simulink model "EMB_Lost_full"  (R2022a)
settings: Solver=VariableStepAuto  StartTime=0.0  StopTime=2  RelTol=1e-3
libraries: slpidlib x24, spsDCVoltageSourceLib x4, spsPermanentMagnetSynchronousMachineLib x4, spsSVPWMGenerator2LevelLib x4, spsUniversalBridgeLib x4, spsdq0toAlphaBetaZeroLib x4, spspowerguiLib x4
(part 1 of 3)
settings Model: SimulationMode=accelerator  Creator=pc  LastModifiedBy=pc

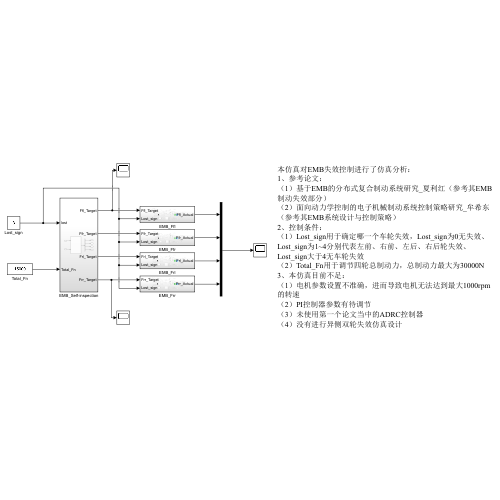
[thumbnail: Simulink's stored preview of the top-level diagram]
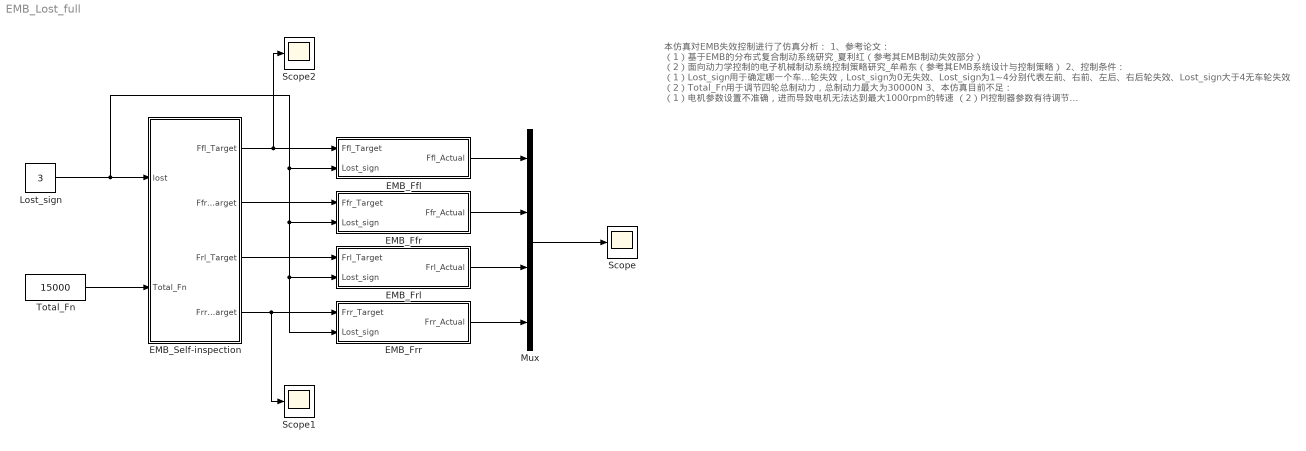
== system EMB_Lost_full ==
  note: 本仿真对EMB失效控制进行了仿真分析：
      | 1、参考论文：
      | （1）基于EMB的分布式复合制动系统研究_夏利红（参考其EMB制动失效部分）
      | （2）面向动力学控制的电子机械制动系统控制策略研究_牟希东（参考其EMB系统设计与控制策略）
      | 2、控制条件：
      | （1）Lost_sign用于确定哪一个车轮失效，Lost_sign为0无失效、Lost_sign为1~4分别代表左前、右前、左后、右后轮失效、Lost_sign大于4无车轮失效
      | （2）Total_Fn用于调节四轮总制动力，总制动力最大为30000N
      | 3、本仿真目前不足：
      | （1）电机参数设置不准确，进而导致电机无法达到最大1000rpm的转速
      | （2）PI控制器参数有待调节
      | （3）未使用第一个论文当中的ADRC控制器
      | （4）没有进行异侧双轮失效仿真设计
  EMB_Ffl : Subsystem
  EMB_Ffr : Subsystem
  EMB_Frl : Subsystem
  EMB_Frr : Subsystem
  EMB_Self-inspection : Subsystem
  Lost_sign : Constant  Value=3
  Mux : Mux
  Scope : Scope
  Scope1 : Scope
  Scope2 : Scope
  Total_Fn : Constant  Value=15000
  wires:
  Total_Fn/1 -> EMB_Self-inspection/2(Total_Fn)
  EMB_Ffl/1(Ffl_Actual) -> Mux/1
  EMB_Ffr/1(Ffr_Actual) -> Mux/2
  EMB_Frl/1(Frl_Actual) -> Mux/3
  EMB_Frr/1(Frr_Actual) -> Mux/4
  Mux/1 -> Scope/1
  EMB_Self-inspection/2(Ffr_Target) -> EMB_Ffr/1(Ffr_Target)
  EMB_Self-inspection/4(Frr_Target) -> Scope1/1, EMB_Frr/1(Frr_Target)
  EMB_Self-inspection/1(Ffl_Target) -> Scope2/1, EMB_Ffl/1(Ffl_Target)
  EMB_Self-inspection/3(Frl_Target) -> EMB_Frl/1(Frl_Target)
  Lost_sign/1 -> EMB_Frr/2(Lost_sign), EMB_Frl/2(Lost_sign), EMB_Ffr/2(Lost_sign), EMB_Ffl/2(Lost_sign), EMB_Self-inspection/1(lost)

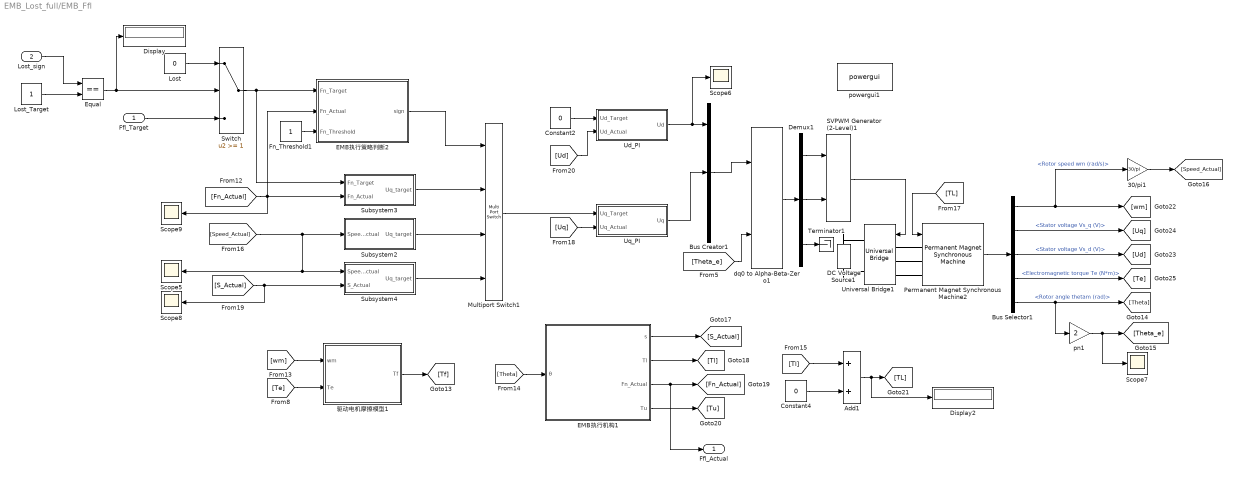
== system EMB_Lost_full/EMB_Ffl ==
  Ffl_Target : Inport
  Lost_sign : Inport  Port=2
  30/pi1 : Gain  Gain=30/pi
  Add1 : Sum
  Bus Creator1 : BusCreator  Inputs=3
  Bus Selector1 : BusSelector  OutputSignals=Rotor speed wm (rad/s),Stator voltage Vs_q (V),Stator voltage Vs_d (V),Electromagnetic torque Te (N*m),Rotor angle thetam (rad)
  Constant2 : Constant  Value=0
  Constant4 : Constant  Value=0
  DC Voltage Source1 : spsDCVoltageSourceLib/DC Voltage Source  Amplitude=24  Measurements=Voltage
  Demux1 : Demux  Outputs=3
  Display : Display
  Display2 : Display
  EMB执行机构1 : Subsystem
  EMB执行策略判断2 : Subsystem
  Equal : RelationalOperator  Operator===  OutDataTypeStr=boolean  RndMeth=Simplest  InputSameDT=off
  Fn_Threshold1 : Constant
  Lost : Constant  Value=0
  Lost_Target : Constant
  Multiport Switch1 : MultiPortSwitch  DiagnosticForDefault=None  SaturateOnIntegerOverflow=off  InputSameDT=off
  Permanent Magnet Synchronous Machine2 : spsPermanentMagnetSynchronousMachineLib/Permanent Magnet Synchronous Machine  NbPhases=3  FluxDistribution=Sinusoidal  RotorType=Round  MechanicalLoad=Torque Tm  PresetModel=No  ShowDetailedParameters=on  MeasurementBus=off  Resistance=1.2  Inductance=8.5e-3  dqInductances=[8.5e-3,8.5e-3]  La=0.0011  MachineConstant=Torque Constant (N.m / A_peak)  Flux=0.072163  VoltageCst=26.178  TorqueCst=0.21649  Flat=120  Mechanical=[9.77*10^-5 0 2 0]  PolePairs=2  InitialConditions=[0,0, 0,0]  InitialConditions5ph=[0 0 0 0 0 0]  RefAngle=90 degrees behind phase A axis (modified Park)  IterativeDiscreteModel=Trapezoidal non iterative  TsBlock=-1  TsPowergui=0
  SVPWM Generator (2-Level)1 : spsSVPWMGenerator2LevelLib/SVPWM Generator (2-Level)  InputType=alpha-beta components  SwitchingPattern=Pattern #1  Fc=2000  ParUref=[0.8 -30 50]  Ts=0
      settings: SourceProductBaseCode=PS
  Scope{5..9} (5 alike) : Scope
  Subsystem2 : Subsystem
  Subsystem3 : Subsystem
  Subsystem4 : Subsystem
  Switch : Switch  Threshold=1  SaturateOnIntegerOverflow=off  InputSameDT=off
  Terminator1 : Terminator
  Ud_PI : Subsystem
  Universal Bridge1 : spsUniversalBridgeLib/Universal Bridge  Arms=3  SnubberResistance=1e5  SnubberCapacitance=inf  Device=IGBT / Diodes  Ron=1e-3  Lon=0  ForwardVoltages="[  0  0  ]"  ForwardVoltage=0  GTOparameters=[ 10e-6 , 20e-6 ]  IGBTparameters=[ 1e-6 , 2e-6 ]  Measurements=None  Measurements_2=None  converterType=Rectifier
  Uq_PI : Subsystem
  dq0 to Alpha-Beta-Zero1 : spsdq0toAlphaBetaZeroLib/dq0 to Alpha-Beta-Zero  Alignment=90 degrees behind phase A axis
      settings: SourceProductBaseCode=PS
  pn1 : Gain  Gain=2
  powergui1 : spspowerguiLib/powergui  Priority=1  SimulationMode=Discrete  SampleTime=5e-7  frequency=60  Iterations=50  frequencyindice=0  Pbase=100e6  ErrMax=1e-4  UnitsV=kV  UnitsW=MW  buscounter=0  FunctionMessages=off  echomessages=off  EnableUseOfTLC=off  CurrentSourceSwitches=off  DisableSnubberDevices=off  DisableRonSwitches=off  DisableVfSwitches=off  DisplayEquations=off  AutomaticDiscreteSolvers=off  SolverType=Tustin/Backward Euler (TBE)  Interpol=off  ExternalGateDelay=off  methode=off  Ts=100  x0status=blocks  SPID=on  SwTol=0  HookPort=off  NonlinearTolerance=1e-4  nMaxIteration=100  ContinueOnMaxIteration=off  RestoreLinks=warning  ResistiveCurrentMeasurement=off  Frange=[0:2:500]  Ylog=off  Xlog=on  ShowGrid=off  save=off  variable=ZData  structure=0  ZoomFFT=off  StartTime=0.0  cycles=1  DisplayStyle=1  fundamental=60  FreqAxis=off  MaxFrequency=1000  frequencyindicesteady=1  RmsSteady=1  display=off
  驱动电机摩擦模型1 : Subsystem
  Ffl_Actual : Outport
  wires:
  Subsystem2/1(Uq_target) -> Multiport Switch1/3
  SVPWM Generator (2-Level)1/1 -> Universal Bridge1/1
  Subsystem4/1(Uq_target) -> Multiport Switch1/4
  Bus Selector1/5 -> pn1/1, [Theta]  "<Rotor angle thetam (rad)>"
  Fn_Threshold1/1 -> EMB执行策略判断2/3(Fn_Threshold)
  [Theta] -> EMB执行机构1/1(θ)
  [Tl] -> Add1/1
  EMB执行机构1/1(s) -> [S_Actual]
  EMB执行机构1/4(Tu) -> [Tu]
  [S_Actual] -> Scope8/1, Subsystem4/2(S_Actual)
  Constant2/1 -> Ud_PI/1(Ud_Target)
  Permanent Magnet Synchronous Machine2/1 -> Bus Selector1/1
  Uq_PI/1(Uq) -> Bus Creator1/2
  Demux1/1 -> SVPWM Generator (2-Level)1/1
  [Fn_Actual] -> Scope9/1, EMB执行策略判断2/2(Fn_Actual), Subsystem3/2(Fn_Actual)
  Bus Creator1/1 -> dq0 to Alpha-Beta-Zero1/1
  [Theta_e] -> dq0 to Alpha-Beta-Zero1/2
  [Ud] -> Ud_PI/2(Ud_Actual)
  [wm] -> 驱动电机摩擦模型1/1(wm)
  Constant4/1 -> Add1/2
  Bus Selector1/3 -> [Ud]  "<Stator voltage Vs_d (V)>"
  Add1/1 -> Display2/1, [TL]
  Multiport Switch1/1 -> Uq_PI/1(Uq_Target)
  [Uq] -> Uq_PI/2(Uq_Actual)
  EMB执行机构1/3(Fn_Actual) -> Ffl_Actual/1, [Fn_Actual]
  Bus Selector1/2 -> [Uq]  "<Stator voltage Vs_q (V)>"
  dq0 to Alpha-Beta-Zero1/1 -> Demux1/1
  [TL] -> Permanent Magnet Synchronous Machine2/1
  [Te] -> 驱动电机摩擦模型1/2(Te)
  驱动电机摩擦模型1/1(Tf) -> [Tf]
  EMB执行策略判断2/1(sign) -> Multiport Switch1/1
  Demux1/3 -> Terminator1/1
  Demux1/2 -> SVPWM Generator (2-Level)1/2
  [Speed_Actual] -> Subsystem2/1(Speed_Actual), Subsystem4/1(Speed_Actual), Scope5/1
  30/pi1/1 -> [Speed_Actual]
  pn1/1 -> Scope7/1, [Theta_e]
  Bus Selector1/4 -> [Te]  "<Electromagnetic torque Te (N*m)>"
  Subsystem3/1(Uq_target) -> Multiport Switch1/2
  Ud_PI/1(Ud) -> Scope6/1, Bus Creator1/1
  EMB执行机构1/2(Tl) -> [Tl]
  Bus Selector1/1 -> [wm], 30/pi1/1  "<Rotor speed wm (rad/s)>"
  Ffl_Target/1 -> Switch/3
  Lost/1 -> Switch/1
  Switch/1 -> EMB执行策略判断2/1(Fn_Target), Subsystem3/1(Fn_Target)
  Lost_sign/1 -> Equal/1
  Equal/1 -> Display/1, Switch/2
  Lost_Target/1 -> Equal/2
  connections:
  DC Voltage Source1/RConn1 -- Universal Bridge1/RConn1
  Permanent Magnet Synchronous Machine2/LConn2 -- Universal Bridge1/LConn2
  Permanent Magnet Synchronous Machine2/LConn1 -- Universal Bridge1/LConn1
  Permanent Magnet Synchronous Machine2/LConn3 -- Universal Bridge1/LConn3
  DC Voltage Source1/LConn1 -- Universal Bridge1/RConn2

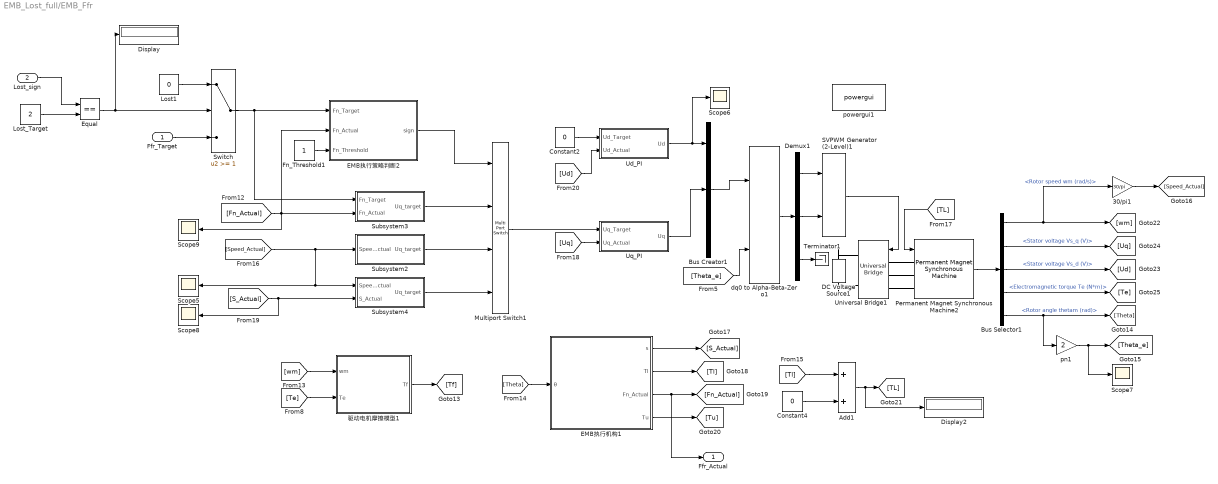
== system EMB_Lost_full/EMB_Ffr ==
  Ffr_Target : Inport
  Lost_sign : Inport  Port=2
  30/pi1 : Gain  Gain=30/pi
  Add1 : Sum
  Bus Creator1 : BusCreator  Inputs=3
  Bus Selector1 : BusSelector  OutputSignals=Rotor speed wm (rad/s),Stator voltage Vs_q (V),Stator voltage Vs_d (V),Electromagnetic torque Te (N*m),Rotor angle thetam (rad)
  Constant2 : Constant  Value=0
  Constant4 : Constant  Value=0
  DC Voltage Source1 : spsDCVoltageSourceLib/DC Voltage Source  Amplitude=24  Measurements=Voltage
  Demux1 : Demux  Outputs=3
  Display : Display
  Display2 : Display
  EMB执行机构1 : Subsystem
  EMB执行策略判断2 : Subsystem
  Equal : RelationalOperator  Operator===  OutDataTypeStr=boolean  RndMeth=Simplest  InputSameDT=off
  Fn_Threshold1 : Constant
  Lost1 : Constant  Value=0
  Lost_Target : Constant  Value=2
  Multiport Switch1 : MultiPortSwitch  DiagnosticForDefault=None  SaturateOnIntegerOverflow=off  InputSameDT=off
  Permanent Magnet Synchronous Machine2 : spsPermanentMagnetSynchronousMachineLib/Permanent Magnet Synchronous Machine  NbPhases=3  FluxDistribution=Sinusoidal  RotorType=Round  MechanicalLoad=Torque Tm  PresetModel=No  ShowDetailedParameters=on  MeasurementBus=off  Resistance=1.2  Inductance=8.5e-3  dqInductances=[8.5e-3,8.5e-3]  La=0.0011  MachineConstant=Torque Constant (N.m / A_peak)  Flux=0.072163  VoltageCst=26.178  TorqueCst=0.21649  Flat=120  Mechanical=[9.77*10^-5 0 2 0]  PolePairs=2  InitialConditions=[0,0, 0,0]  InitialConditions5ph=[0 0 0 0 0 0]  RefAngle=90 degrees behind phase A axis (modified Park)  IterativeDiscreteModel=Trapezoidal non iterative  TsBlock=-1  TsPowergui=0
  SVPWM Generator (2-Level)1 : spsSVPWMGenerator2LevelLib/SVPWM Generator (2-Level)  InputType=alpha-beta components  SwitchingPattern=Pattern #1  Fc=2000  ParUref=[0.8 -30 50]  Ts=0
      settings: SourceProductBaseCode=PS
  Scope{5..9} (5 alike) : Scope
  Subsystem2 : Subsystem
  Subsystem3 : Subsystem
  Subsystem4 : Subsystem
  Switch : Switch  Threshold=1  SaturateOnIntegerOverflow=off  InputSameDT=off
  Terminator1 : Terminator
  Ud_PI : Subsystem
  Universal Bridge1 : spsUniversalBridgeLib/Universal Bridge  Arms=3  SnubberResistance=1e5  SnubberCapacitance=inf  Device=IGBT / Diodes  Ron=1e-3  Lon=0  ForwardVoltages="[  0  0  ]"  ForwardVoltage=0  GTOparameters=[ 10e-6 , 20e-6 ]  IGBTparameters=[ 1e-6 , 2e-6 ]  Measurements=None  Measurements_2=None  converterType=Rectifier
  Uq_PI : Subsystem
  dq0 to Alpha-Beta-Zero1 : spsdq0toAlphaBetaZeroLib/dq0 to Alpha-Beta-Zero  Alignment=90 degrees behind phase A axis
      settings: SourceProductBaseCode=PS
  pn1 : Gain  Gain=2
  powergui1 : spspowerguiLib/powergui  Priority=1  SimulationMode=Discrete  SampleTime=5e-7  frequency=60  Iterations=50  frequencyindice=0  Pbase=100e6  ErrMax=1e-4  UnitsV=kV  UnitsW=MW  buscounter=0  FunctionMessages=off  echomessages=off  EnableUseOfTLC=off  CurrentSourceSwitches=off  DisableSnubberDevices=off  DisableRonSwitches=off  DisableVfSwitches=off  DisplayEquations=off  AutomaticDiscreteSolvers=off  SolverType=Tustin/Backward Euler (TBE)  Interpol=off  ExternalGateDelay=off  methode=off  Ts=100  x0status=blocks  SPID=on  SwTol=0  HookPort=off  NonlinearTolerance=1e-4  nMaxIteration=100  ContinueOnMaxIteration=off  RestoreLinks=warning  ResistiveCurrentMeasurement=off  Frange=[0:2:500]  Ylog=off  Xlog=on  ShowGrid=off  save=off  variable=ZData  structure=0  ZoomFFT=off  StartTime=0.0  cycles=1  DisplayStyle=1  fundamental=60  FreqAxis=off  MaxFrequency=1000  frequencyindicesteady=1  RmsSteady=1  display=off
  驱动电机摩擦模型1 : Subsystem
  Ffr_Actual : Outport
  wires:
  Subsystem2/1(Uq_target) -> Multiport Switch1/3
  SVPWM Generator (2-Level)1/1 -> Universal Bridge1/1
  Subsystem4/1(Uq_target) -> Multiport Switch1/4
  Bus Selector1/5 -> pn1/1, [Theta]  "<Rotor angle thetam (rad)>"
  Fn_Threshold1/1 -> EMB执行策略判断2/3(Fn_Threshold)
  [Theta] -> EMB执行机构1/1(θ)
  [Tl] -> Add1/1
  EMB执行机构1/1(s) -> [S_Actual]
  EMB执行机构1/4(Tu) -> [Tu]
  [S_Actual] -> Scope8/1, Subsystem4/2(S_Actual)
  Constant2/1 -> Ud_PI/1(Ud_Target)
  Permanent Magnet Synchronous Machine2/1 -> Bus Selector1/1
  Uq_PI/1(Uq) -> Bus Creator1/2
  Ffr_Target/1 -> Switch/3
  Demux1/1 -> SVPWM Generator (2-Level)1/1
  [Fn_Actual] -> Scope9/1, EMB执行策略判断2/2(Fn_Actual), Subsystem3/2(Fn_Actual)
  Bus Creator1/1 -> dq0 to Alpha-Beta-Zero1/1
  [Theta_e] -> dq0 to Alpha-Beta-Zero1/2
  [Ud] -> Ud_PI/2(Ud_Actual)
  [wm] -> 驱动电机摩擦模型1/1(wm)
  Constant4/1 -> Add1/2
  Bus Selector1/3 -> [Ud]  "<Stator voltage Vs_d (V)>"
  Add1/1 -> Display2/1, [TL]
  Multiport Switch1/1 -> Uq_PI/1(Uq_Target)
  [Uq] -> Uq_PI/2(Uq_Actual)
  EMB执行机构1/3(Fn_Actual) -> Ffr_Actual/1, [Fn_Actual]
  Bus Selector1/2 -> [Uq]  "<Stator voltage Vs_q (V)>"
  dq0 to Alpha-Beta-Zero1/1 -> Demux1/1
  [TL] -> Permanent Magnet Synchronous Machine2/1
  [Te] -> 驱动电机摩擦模型1/2(Te)
  驱动电机摩擦模型1/1(Tf) -> [Tf]
  EMB执行策略判断2/1(sign) -> Multiport Switch1/1
  Demux1/3 -> Terminator1/1
  Demux1/2 -> SVPWM Generator (2-Level)1/2
  [Speed_Actual] -> Subsystem2/1(Speed_Actual), Subsystem4/1(Speed_Actual), Scope5/1
  30/pi1/1 -> [Speed_Actual]
  pn1/1 -> Scope7/1, [Theta_e]
  Bus Selector1/4 -> [Te]  "<Electromagnetic torque Te (N*m)>"
  Subsystem3/1(Uq_target) -> Multiport Switch1/2
  Ud_PI/1(Ud) -> Scope6/1, Bus Creator1/1
  EMB执行机构1/2(Tl) -> [Tl]
  Bus Selector1/1 -> [wm], 30/pi1/1  "<Rotor speed wm (rad/s)>"
  Switch/1 -> Subsystem3/1(Fn_Target), EMB执行策略判断2/1(Fn_Target)
  Lost1/1 -> Switch/1
  Equal/1 -> Display/1, Switch/2
  Lost_sign/1 -> Equal/1
  Lost_Target/1 -> Equal/2
  connections:
  DC Voltage Source1/RConn1 -- Universal Bridge1/RConn1
  Permanent Magnet Synchronous Machine2/LConn2 -- Universal Bridge1/LConn2
  Permanent Magnet Synchronous Machine2/LConn1 -- Universal Bridge1/LConn1
  Permanent Magnet Synchronous Machine2/LConn3 -- Universal Bridge1/LConn3
  DC Voltage Source1/LConn1 -- Universal Bridge1/RConn2

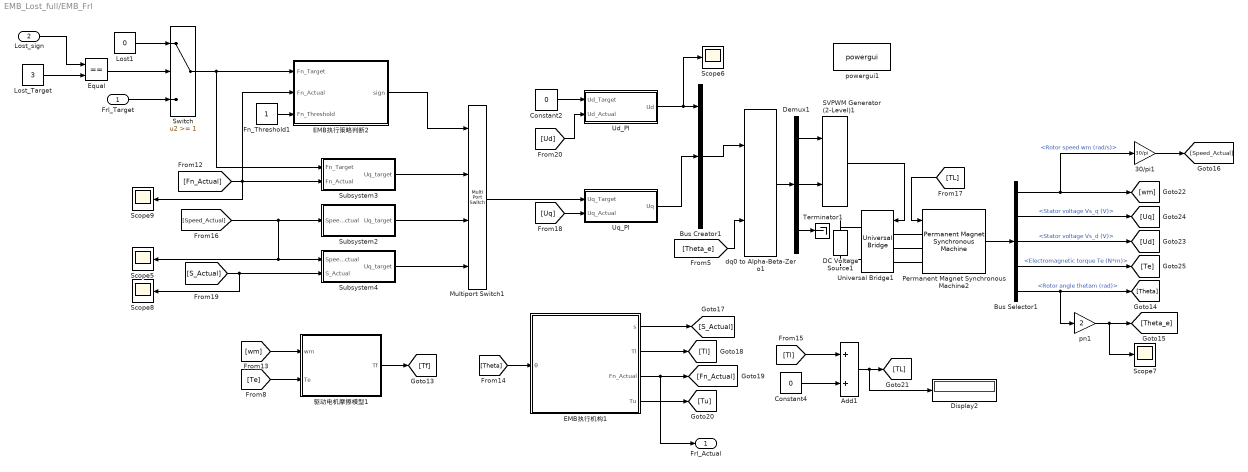
== system EMB_Lost_full/EMB_Frl ==
  Frl_Target : Inport
  Lost_sign : Inport  Port=2
  30/pi1 : Gain  Gain=30/pi
  Add1 : Sum
  Bus Creator1 : BusCreator  Inputs=3
  Bus Selector1 : BusSelector  OutputSignals=Rotor speed wm (rad/s),Stator voltage Vs_q (V),Stator voltage Vs_d (V),Electromagnetic torque Te (N*m),Rotor angle thetam (rad)
  Constant2 : Constant  Value=0
  Constant4 : Constant  Value=0
  DC Voltage Source1 : spsDCVoltageSourceLib/DC Voltage Source  Amplitude=24  Measurements=Voltage
  Demux1 : Demux  Outputs=3
  Display2 : Display
  EMB执行机构1 : Subsystem
  EMB执行策略判断2 : Subsystem
  Equal : RelationalOperator  Operator===  OutDataTypeStr=boolean  RndMeth=Simplest  InputSameDT=off
  Fn_Threshold1 : Constant
  Lost1 : Constant  Value=0
  Lost_Target : Constant  Value=3
  Multiport Switch1 : MultiPortSwitch  DiagnosticForDefault=None  SaturateOnIntegerOverflow=off  InputSameDT=off
  Permanent Magnet Synchronous Machine2 : spsPermanentMagnetSynchronousMachineLib/Permanent Magnet Synchronous Machine  NbPhases=3  FluxDistribution=Sinusoidal  RotorType=Round  MechanicalLoad=Torque Tm  PresetModel=No  ShowDetailedParameters=on  MeasurementBus=off  Resistance=1.2  Inductance=8.5e-3  dqInductances=[8.5e-3,8.5e-3]  La=0.0011  MachineConstant=Torque Constant (N.m / A_peak)  Flux=0.072163  VoltageCst=26.178  TorqueCst=0.21649  Flat=120  Mechanical=[9.77*10^-5 0 2 0]  PolePairs=2  InitialConditions=[0,0, 0,0]  InitialConditions5ph=[0 0 0 0 0 0]  RefAngle=90 degrees behind phase A axis (modified Park)  IterativeDiscreteModel=Trapezoidal non iterative  TsBlock=-1  TsPowergui=0
  SVPWM Generator (2-Level)1 : spsSVPWMGenerator2LevelLib/SVPWM Generator (2-Level)  InputType=alpha-beta components  SwitchingPattern=Pattern #1  Fc=2000  ParUref=[0.8 -30 50]  Ts=0
      settings: SourceProductBaseCode=PS
  Scope{5..9} (5 alike) : Scope
  Subsystem2 : Subsystem
  Subsystem3 : Subsystem
  Subsystem4 : Subsystem
  Switch : Switch  Threshold=1  SaturateOnIntegerOverflow=off  InputSameDT=off
  Terminator1 : Terminator
  Ud_PI : Subsystem
  Universal Bridge1 : spsUniversalBridgeLib/Universal Bridge  Arms=3  SnubberResistance=1e5  SnubberCapacitance=inf  Device=IGBT / Diodes  Ron=1e-3  Lon=0  ForwardVoltages="[  0  0  ]"  ForwardVoltage=0  GTOparameters=[ 10e-6 , 20e-6 ]  IGBTparameters=[ 1e-6 , 2e-6 ]  Measurements=None  Measurements_2=None  converterType=Rectifier
  Uq_PI : Subsystem
  dq0 to Alpha-Beta-Zero1 : spsdq0toAlphaBetaZeroLib/dq0 to Alpha-Beta-Zero  Alignment=90 degrees behind phase A axis
      settings: SourceProductBaseCode=PS
  pn1 : Gain  Gain=2
  powergui1 : spspowerguiLib/powergui  Priority=1  SimulationMode=Discrete  SampleTime=5e-7  frequency=60  Iterations=50  frequencyindice=0  Pbase=100e6  ErrMax=1e-4  UnitsV=kV  UnitsW=MW  buscounter=0  FunctionMessages=off  echomessages=off  EnableUseOfTLC=off  CurrentSourceSwitches=off  DisableSnubberDevices=off  DisableRonSwitches=off  DisableVfSwitches=off  DisplayEquations=off  AutomaticDiscreteSolvers=off  SolverType=Tustin/Backward Euler (TBE)  Interpol=off  ExternalGateDelay=off  methode=off  Ts=100  x0status=blocks  SPID=on  SwTol=0  HookPort=off  NonlinearTolerance=1e-4  nMaxIteration=100  ContinueOnMaxIteration=off  RestoreLinks=warning  ResistiveCurrentMeasurement=off  Frange=[0:2:500]  Ylog=off  Xlog=on  ShowGrid=off  save=off  variable=ZData  structure=0  ZoomFFT=off  StartTime=0.0  cycles=1  DisplayStyle=1  fundamental=60  FreqAxis=off  MaxFrequency=1000  frequencyindicesteady=1  RmsSteady=1  display=off
  驱动电机摩擦模型1 : Subsystem
  Frl_Actual : Outport
  wires:
  Subsystem2/1(Uq_target) -> Multiport Switch1/3
  SVPWM Generator (2-Level)1/1 -> Universal Bridge1/1
  Subsystem4/1(Uq_target) -> Multiport Switch1/4
  Bus Selector1/5 -> pn1/1, [Theta]  "<Rotor angle thetam (rad)>"
  Fn_Threshold1/1 -> EMB执行策略判断2/3(Fn_Threshold)
  [Theta] -> EMB执行机构1/1(θ)
  [Tl] -> Add1/1
  EMB执行机构1/1(s) -> [S_Actual]
  EMB执行机构1/4(Tu) -> [Tu]
  [S_Actual] -> Scope8/1, Subsystem4/2(S_Actual)
  Constant2/1 -> Ud_PI/1(Ud_Target)
  Permanent Magnet Synchronous Machine2/1 -> Bus Selector1/1
  Uq_PI/1(Uq) -> Bus Creator1/2
  Demux1/1 -> SVPWM Generator (2-Level)1/1
  [Fn_Actual] -> Scope9/1, EMB执行策略判断2/2(Fn_Actual), Subsystem3/2(Fn_Actual)
  Bus Creator1/1 -> dq0 to Alpha-Beta-Zero1/1
  [Theta_e] -> dq0 to Alpha-Beta-Zero1/2
  [Ud] -> Ud_PI/2(Ud_Actual)
  [wm] -> 驱动电机摩擦模型1/1(wm)
  Constant4/1 -> Add1/2
  Bus Selector1/3 -> [Ud]  "<Stator voltage Vs_d (V)>"
  Add1/1 -> Display2/1, [TL]
  Multiport Switch1/1 -> Uq_PI/1(Uq_Target)
  [Uq] -> Uq_PI/2(Uq_Actual)
  EMB执行机构1/3(Fn_Actual) -> Frl_Actual/1, [Fn_Actual]
  Bus Selector1/2 -> [Uq]  "<Stator voltage Vs_q (V)>"
  dq0 to Alpha-Beta-Zero1/1 -> Demux1/1
  [TL] -> Permanent Magnet Synchronous Machine2/1
  [Te] -> 驱动电机摩擦模型1/2(Te)
  驱动电机摩擦模型1/1(Tf) -> [Tf]
  EMB执行策略判断2/1(sign) -> Multiport Switch1/1
  Demux1/3 -> Terminator1/1
  Demux1/2 -> SVPWM Generator (2-Level)1/2
  [Speed_Actual] -> Subsystem2/1(Speed_Actual), Subsystem4/1(Speed_Actual), Scope5/1
  30/pi1/1 -> [Speed_Actual]
  pn1/1 -> Scope7/1, [Theta_e]
  Bus Selector1/4 -> [Te]  "<Electromagnetic torque Te (N*m)>"
  Subsystem3/1(Uq_target) -> Multiport Switch1/2
  Ud_PI/1(Ud) -> Scope6/1, Bus Creator1/1
  EMB执行机构1/2(Tl) -> [Tl]
  Bus Selector1/1 -> [wm], 30/pi1/1  "<Rotor speed wm (rad/s)>"
  Switch/1 -> Subsystem3/1(Fn_Target), EMB执行策略判断2/1(Fn_Target)
  Frl_Target/1 -> Switch/3
  Lost1/1 -> Switch/1
  Lost_sign/1 -> Equal/1
  Equal/1 -> Switch/2
  Lost_Target/1 -> Equal/2
  connections:
  DC Voltage Source1/RConn1 -- Universal Bridge1/RConn1
  Permanent Magnet Synchronous Machine2/LConn2 -- Universal Bridge1/LConn2
  Permanent Magnet Synchronous Machine2/LConn1 -- Universal Bridge1/LConn1
  Permanent Magnet Synchronous Machine2/LConn3 -- Universal Bridge1/LConn3
  DC Voltage Source1/LConn1 -- Universal Bridge1/RConn2

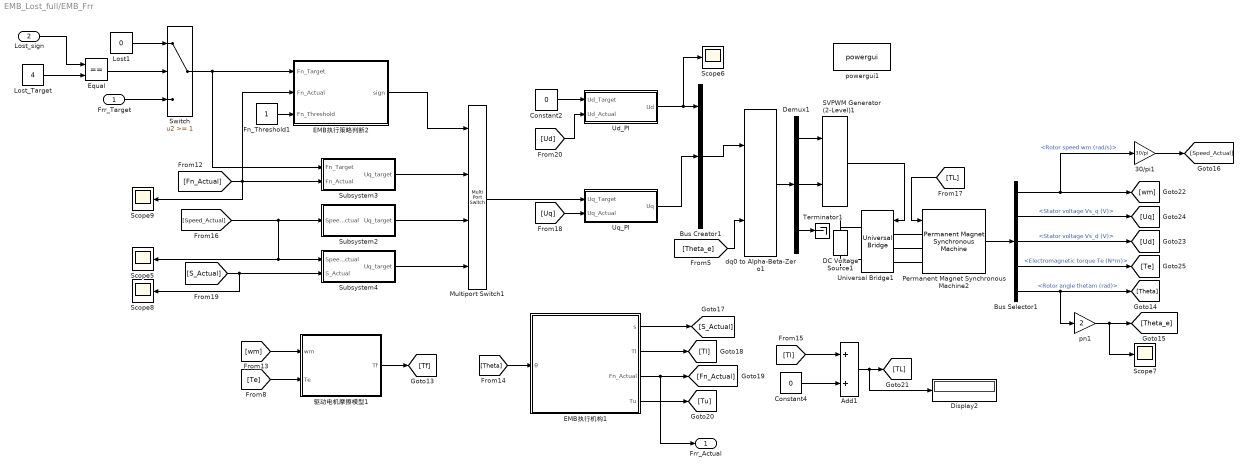
== system EMB_Lost_full/EMB_Frr ==
  Frr_Target : Inport
  Lost_sign : Inport  Port=2
  30/pi1 : Gain  Gain=30/pi
  Add1 : Sum
  Bus Creator1 : BusCreator  Inputs=3
  Bus Selector1 : BusSelector  OutputSignals=Rotor speed wm (rad/s),Stator voltage Vs_q (V),Stator voltage Vs_d (V),Electromagnetic torque Te (N*m),Rotor angle thetam (rad)
  Constant2 : Constant  Value=0
  Constant4 : Constant  Value=0
  DC Voltage Source1 : spsDCVoltageSourceLib/DC Voltage Source  Amplitude=24  Measurements=Voltage
  Demux1 : Demux  Outputs=3
  Display2 : Display
  EMB执行机构1 : Subsystem
  EMB执行策略判断2 : Subsystem
  Equal : RelationalOperator  Operator===  OutDataTypeStr=boolean  RndMeth=Simplest  InputSameDT=off
  Fn_Threshold1 : Constant
  Lost1 : Constant  Value=0
  Lost_Target : Constant  Value=4
  Multiport Switch1 : MultiPortSwitch  DiagnosticForDefault=None  SaturateOnIntegerOverflow=off  InputSameDT=off
  Permanent Magnet Synchronous Machine2 : spsPermanentMagnetSynchronousMachineLib/Permanent Magnet Synchronous Machine  NbPhases=3  FluxDistribution=Sinusoidal  RotorType=Round  MechanicalLoad=Torque Tm  PresetModel=No  ShowDetailedParameters=on  MeasurementBus=off  Resistance=1.2  Inductance=8.5e-3  dqInductances=[8.5e-3,8.5e-3]  La=0.0011  MachineConstant=Torque Constant (N.m / A_peak)  Flux=0.072163  VoltageCst=26.178  TorqueCst=0.21649  Flat=120  Mechanical=[9.77*10^-5 0 2 0]  PolePairs=2  InitialConditions=[0,0, 0,0]  InitialConditions5ph=[0 0 0 0 0 0]  RefAngle=90 degrees behind phase A axis (modified Park)  IterativeDiscreteModel=Trapezoidal non iterative  TsBlock=-1  TsPowergui=0
  SVPWM Generator (2-Level)1 : spsSVPWMGenerator2LevelLib/SVPWM Generator (2-Level)  InputType=alpha-beta components  SwitchingPattern=Pattern #1  Fc=2000  ParUref=[0.8 -30 50]  Ts=0
      settings: SourceProductBaseCode=PS
  Scope{5..9} (5 alike) : Scope
  Subsystem2 : Subsystem
  Subsystem3 : Subsystem
  Subsystem4 : Subsystem
  Switch : Switch  Threshold=1  SaturateOnIntegerOverflow=off  InputSameDT=off
  Terminator1 : Terminator
  Ud_PI : Subsystem
  Universal Bridge1 : spsUniversalBridgeLib/Universal Bridge  Arms=3  SnubberResistance=1e5  SnubberCapacitance=inf  Device=IGBT / Diodes  Ron=1e-3  Lon=0  ForwardVoltages="[  0  0  ]"  ForwardVoltage=0  GTOparameters=[ 10e-6 , 20e-6 ]  IGBTparameters=[ 1e-6 , 2e-6 ]  Measurements=None  Measurements_2=None  converterType=Rectifier
  Uq_PI : Subsystem
  dq0 to Alpha-Beta-Zero1 : spsdq0toAlphaBetaZeroLib/dq0 to Alpha-Beta-Zero  Alignment=90 degrees behind phase A axis
      settings: SourceProductBaseCode=PS
  pn1 : Gain  Gain=2
  powergui1 : spspowerguiLib/powergui  Priority=1  SimulationMode=Discrete  SampleTime=5e-7  frequency=60  Iterations=50  frequencyindice=0  Pbase=100e6  ErrMax=1e-4  UnitsV=kV  UnitsW=MW  buscounter=0  FunctionMessages=off  echomessages=off  EnableUseOfTLC=off  CurrentSourceSwitches=off  DisableSnubberDevices=off  DisableRonSwitches=off  DisableVfSwitches=off  DisplayEquations=off  AutomaticDiscreteSolvers=off  SolverType=Tustin/Backward Euler (TBE)  Interpol=off  ExternalGateDelay=off  methode=off  Ts=100  x0status=blocks  SPID=on  SwTol=0  HookPort=off  NonlinearTolerance=1e-4  nMaxIteration=100  ContinueOnMaxIteration=off  RestoreLinks=warning  ResistiveCurrentMeasurement=off  Frange=[0:2:500]  Ylog=off  Xlog=on  ShowGrid=off  save=off  variable=ZData  structure=0  ZoomFFT=off  StartTime=0.0  cycles=1  DisplayStyle=1  fundamental=60  FreqAxis=off  MaxFrequency=1000  frequencyindicesteady=1  RmsSteady=1  display=off
  驱动电机摩擦模型1 : Subsystem
  Frr_Actual : Outport
  wires:
  Subsystem2/1(Uq_target) -> Multiport Switch1/3
  SVPWM Generator (2-Level)1/1 -> Universal Bridge1/1
  Subsystem4/1(Uq_target) -> Multiport Switch1/4
  Bus Selector1/5 -> pn1/1, [Theta]  "<Rotor angle thetam (rad)>"
  Fn_Threshold1/1 -> EMB执行策略判断2/3(Fn_Threshold)
  [Theta] -> EMB执行机构1/1(θ)
  [Tl] -> Add1/1
  EMB执行机构1/1(s) -> [S_Actual]
  EMB执行机构1/4(Tu) -> [Tu]
  [S_Actual] -> Scope8/1, Subsystem4/2(S_Actual)
  Constant2/1 -> Ud_PI/1(Ud_Target)
  Permanent Magnet Synchronous Machine2/1 -> Bus Selector1/1
  Uq_PI/1(Uq) -> Bus Creator1/2
  Demux1/1 -> SVPWM Generator (2-Level)1/1
  [Fn_Actual] -> Scope9/1, EMB执行策略判断2/2(Fn_Actual), Subsystem3/2(Fn_Actual)
  Bus Creator1/1 -> dq0 to Alpha-Beta-Zero1/1
  [Theta_e] -> dq0 to Alpha-Beta-Zero1/2
  [Ud] -> Ud_PI/2(Ud_Actual)
  [wm] -> 驱动电机摩擦模型1/1(wm)
  Constant4/1 -> Add1/2
  Bus Selector1/3 -> [Ud]  "<Stator voltage Vs_d (V)>"
  Add1/1 -> Display2/1, [TL]
  Multiport Switch1/1 -> Uq_PI/1(Uq_Target)
  [Uq] -> Uq_PI/2(Uq_Actual)
  EMB执行机构1/3(Fn_Actual) -> Frr_Actual/1, [Fn_Actual]
  Bus Selector1/2 -> [Uq]  "<Stator voltage Vs_q (V)>"
  dq0 to Alpha-Beta-Zero1/1 -> Demux1/1
  [TL] -> Permanent Magnet Synchronous Machine2/1
  [Te] -> 驱动电机摩擦模型1/2(Te)
  驱动电机摩擦模型1/1(Tf) -> [Tf]
  EMB执行策略判断2/1(sign) -> Multiport Switch1/1
  Demux1/3 -> Terminator1/1
  Demux1/2 -> SVPWM Generator (2-Level)1/2
  [Speed_Actual] -> Subsystem2/1(Speed_Actual), Subsystem4/1(Speed_Actual), Scope5/1
  30/pi1/1 -> [Speed_Actual]
  pn1/1 -> Scope7/1, [Theta_e]
  Bus Selector1/4 -> [Te]  "<Electromagnetic torque Te (N*m)>"
  Subsystem3/1(Uq_target) -> Multiport Switch1/2
  Ud_PI/1(Ud) -> Scope6/1, Bus Creator1/1
  EMB执行机构1/2(Tl) -> [Tl]
  Bus Selector1/1 -> [wm], 30/pi1/1  "<Rotor speed wm (rad/s)>"
  Frr_Target/1 -> Switch/3
  Equal/1 -> Switch/2
  Lost1/1 -> Switch/1
  Switch/1 -> Subsystem3/1(Fn_Target), EMB执行策略判断2/1(Fn_Target)
  Lost_sign/1 -> Equal/1
  Lost_Target/1 -> Equal/2
  connections:
  DC Voltage Source1/RConn1 -- Universal Bridge1/RConn1
  Permanent Magnet Synchronous Machine2/LConn2 -- Universal Bridge1/LConn2
  Permanent Magnet Synchronous Machine2/LConn1 -- Universal Bridge1/LConn1
  Permanent Magnet Synchronous Machine2/LConn3 -- Universal Bridge1/LConn3
  DC Voltage Source1/LConn1 -- Universal Bridge1/RConn2

== system EMB_Lost_full/EMB_Self-inspection ==
  lost : Inport
  Total_Fn : Inport  Port=2
  Demux1 : Demux
  MATLAB Function : MATLAB Function  TreatAsAtomicUnit=on
  Ffl_Target : Outport
  Ffr_Target : Outport  Port=2
  Frl_Target : Outport  Port=3
  Frr_Target : Outport  Port=4
  wires:
  Total_Fn/1 -> MATLAB Function/1(Total_Fn)
  lost/1 -> MATLAB Function/2(lost)
  MATLAB Function/1(Fn_Target) -> Demux1/1
  Demux1/1 -> Ffl_Target/1
  Demux1/2 -> Ffr_Target/1
  Demux1/3 -> Frl_Target/1
  Demux1/4 -> Frr_Target/1

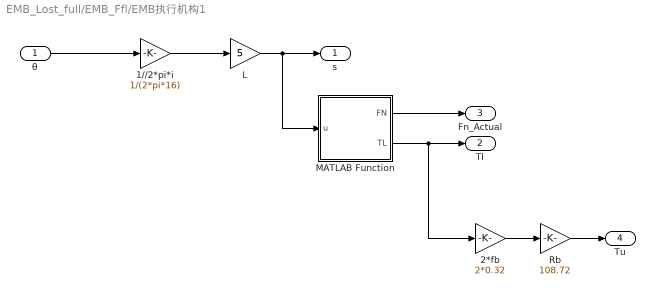
== system EMB_Lost_full/EMB_Ffl/EMB执行机构1 ==
  θ : Inport
  1//2*pi*i : Gain  Gain=1/(2*pi*16)
  2*fb : Gain  Gain=2*0.32
  L : Gain  Gain=5
  MATLAB Function : MATLAB Function  TreatAsAtomicUnit=on
  Rb : Gain  Gain=108.72
  s : Outport
  Tl : Outport  Port=2
  Fn_Actual : Outport  Port=3
  Tu : Outport  Port=4
  wires:
  θ/1 -> 1//2*pi*i/1
  1//2*pi*i/1 -> L/1
  L/1 -> MATLAB Function/1(u), s/1
  MATLAB Function/2(TL) -> 2*fb/1, Tl/1
  MATLAB Function/1(FN) -> Fn_Actual/1
  Rb/1 -> Tu/1
  2*fb/1 -> Rb/1

== system EMB_Lost_full/EMB_Ffl/EMB执行策略判断2 ==
  Fn_Target : Inport
  Fn_Actual : Inport  Port=2
  Fn_Threshold : Inport  Port=3
  MATLAB Function : MATLAB Function  TreatAsAtomicUnit=on
  sign : Outport
  wires:
  Fn_Target/1 -> MATLAB Function/1(Fn_Target)
  Fn_Actual/1 -> MATLAB Function/2(Fn_Actual)
  Fn_Threshold/1 -> MATLAB Function/3(Fn_Threshold)
  MATLAB Function/1(y) -> sign/1

== system EMB_Lost_full/EMB_Ffl/Subsystem2 ==
  Speed_Actual : Inport
  PID Controller : slpidlib/PID Controller  Controller=PI  Form=Parallel  TimeDomain=Continuous-time  UseExternalTs=off  SampleTime=-1  IntegratorMethod=Forward Euler  FilterMethod=Forward Euler  ControllerParametersSource=internal  P=1000  I=0  UseKiTs=off  D=0  N=100  UseFilter=on  TunerSelectOption=Transfer Function Based (PID Tuner App)  InitialConditionSource=internal  InitialConditionForIntegrator=0  InitialConditionForFilter=0  DifferentiatorICPrevScaledInput=0  ExternalReset=none  TrackingMode=off  Kt=1  LimitOutput=on  SatLimitsSource=internal  UpperSaturationLimit=24  LowerSaturationLimit=-24  LinearizeAsGain=on  AntiWindupMode=none  Kb=1  POutMin=[]  POutMax=[]  IOutMin=[]  IOutMax=[]  DOutMin=[]  DOutMax=[]  NOutMin=[]  NOutMax=[]  SumOutMin=[]  SumOutMax=[]  SaturationOutMin=[]  SaturationOutMax=[]  PParamMin=[]  PParamMax=[]  IParamMin=[]  IParamMax=[]  DParamMin=[]  DParamMax=[]  NParamMin=[]  NParamMax=[]  KbParamMin=[]  KbParamMax=[]  KtParamMin=[]  KtParamMax=[]  KbOutMin=[]  KbOutMax=[]  KtOutMin=[]  KtOutMax=[]  IntegratorOutMin=[]  IntegratorOutMax=[]  FilterOutMin=[]  FilterOutMax=[]  SumI1OutMin=[]  SumI1OutMax=[]  SumI2OutMin=[]  SumI2OutMax=[]  SumI3OutMin=[]  SumI3OutMax=[]  SumI4OutMin=[]  SumI4OutMax=[]  SumDOutMin=[]  SumDOutMax=[]  DifferentiatorOutMin=[]  DifferentiatorOutMax=[]  FilterDiffOutCoefMin=[]  FilterDiffOutCoefMax=[]  ReciprocalOutMin=[]  ReciprocalOutMax=[]  SumDenOutMin=[]  SumDenOutMax=[]  SumNumOutMin=[]  SumNumOutMax=[]  DivideOutMin=[]  DivideOutMax=[]  UdiffTsProdOutMin=[]  UdiffTsProdOutMax=[]  NTsProdOutMin=[]  NTsProdOutMax=[]  UintegralTsProdOutMin=[]  UintegralTsProdOutMax=[]  UngainTsProdOutMin=[]  UngainTsProdOutMax=[]  IntegratorContinuousStateAttributes=''  IntegratorStateMustResolveToSignalObject=off  IntegratorRTWStateStorageClass=Auto  FilterContinuousStateAttributes=''  FilterStateMustResolveToSignalObject=off  FilterRTWStateStorageClass=Auto  ParallelPVariant=InternalParameters  IdealPVariant=Disabled  IVariant=InternalParameters  DVariant=Disabled  IntegratorVariant=Continuous  SatVariant=Enabled  AWVariant=Passthrough  PCopyVariant=Disabled  TRVariant=Disabled  FdbkBlocksVariant=Forward  IdealPFdbkVariant=Disabled  SatFdbkVariant=Disabled  DerivativeFilterVariant=Disabled  NVariant=Disabled  NCopyVariant=Disabled_SignalSpec  FilterICVariant=Disabled  IntegratorICVariant=InternalICs  ExternalResetVariant=Disabled  TRSumVariant=Passthrough  SumFdbkVariant=Disabled  SumVariant=Sum_PI  TsampFilterVariant=InternalTs  TsampNgainVariant=Passthrough  TsampIntegralVariant=Passthrough  ExternalSaturationOutDataTypeStr=Inherit: Same as second input  aMode=0
  Speed_Target : Constant  Value=1000
  Sum : Sum  Inputs=|+-
  Uq_target : Outport
  wires:
  Speed_Target/1 -> Sum/1
  Sum/1 -> PID Controller/1
  PID Controller/1 -> Uq_target/1
  Speed_Actual/1 -> Sum/2

== system EMB_Lost_full/EMB_Ffl/Subsystem3 ==
  Fn_Target : Inport
  Fn_Actual : Inport  Port=2
  PID Controller : slpidlib/PID Controller  Controller=PI  Form=Parallel  TimeDomain=Continuous-time  UseExternalTs=off  SampleTime=-1  IntegratorMethod=Forward Euler  FilterMethod=Forward Euler  ControllerParametersSource=internal  P=0.08  I=0  UseKiTs=off  D=0  N=100  UseFilter=on  TunerSelectOption=Transfer Function Based (PID Tuner App)  InitialConditionSource=internal  InitialConditionForIntegrator=0  InitialConditionForFilter=0  DifferentiatorICPrevScaledInput=0  ExternalReset=none  TrackingMode=off  Kt=1  LimitOutput=on  SatLimitsSource=internal  UpperSaturationLimit=24  LowerSaturationLimit=-24  LinearizeAsGain=on  AntiWindupMode=none  Kb=1  POutMin=[]  POutMax=[]  IOutMin=[]  IOutMax=[]  DOutMin=[]  DOutMax=[]  NOutMin=[]  NOutMax=[]  SumOutMin=[]  SumOutMax=[]  SaturationOutMin=[]  SaturationOutMax=[]  PParamMin=[]  PParamMax=[]  IParamMin=[]  IParamMax=[]  DParamMin=[]  DParamMax=[]  NParamMin=[]  NParamMax=[]  KbParamMin=[]  KbParamMax=[]  KtParamMin=[]  KtParamMax=[]  KbOutMin=[]  KbOutMax=[]  KtOutMin=[]  KtOutMax=[]  IntegratorOutMin=[]  IntegratorOutMax=[]  FilterOutMin=[]  FilterOutMax=[]  SumI1OutMin=[]  SumI1OutMax=[]  SumI2OutMin=[]  SumI2OutMax=[]  SumI3OutMin=[]  SumI3OutMax=[]  SumI4OutMin=[]  SumI4OutMax=[]  SumDOutMin=[]  SumDOutMax=[]  DifferentiatorOutMin=[]  DifferentiatorOutMax=[]  FilterDiffOutCoefMin=[]  FilterDiffOutCoefMax=[]  ReciprocalOutMin=[]  ReciprocalOutMax=[]  SumDenOutMin=[]  SumDenOutMax=[]  SumNumOutMin=[]  SumNumOutMax=[]  DivideOutMin=[]  DivideOutMax=[]  UdiffTsProdOutMin=[]  UdiffTsProdOutMax=[]  NTsProdOutMin=[]  NTsProdOutMax=[]  UintegralTsProdOutMin=[]  UintegralTsProdOutMax=[]  UngainTsProdOutMin=[]  UngainTsProdOutMax=[]  IntegratorContinuousStateAttributes=''  IntegratorStateMustResolveToSignalObject=off  IntegratorRTWStateStorageClass=Auto  FilterContinuousStateAttributes=''  FilterStateMustResolveToSignalObject=off  FilterRTWStateStorageClass=Auto  ParallelPVariant=InternalParameters  IdealPVariant=Disabled  IVariant=InternalParameters  DVariant=Disabled  IntegratorVariant=Continuous  SatVariant=Enabled  AWVariant=Passthrough  PCopyVariant=Disabled  TRVariant=Disabled  FdbkBlocksVariant=Forward  IdealPFdbkVariant=Disabled  SatFdbkVariant=Disabled  DerivativeFilterVariant=Disabled  NVariant=Disabled  NCopyVariant=Disabled_SignalSpec  FilterICVariant=Disabled  IntegratorICVariant=InternalICs  ExternalResetVariant=Disabled  TRSumVariant=Passthrough  SumFdbkVariant=Disabled  SumVariant=Sum_PI  TsampFilterVariant=InternalTs  TsampNgainVariant=Passthrough  TsampIntegralVariant=Passthrough  ExternalSaturationOutDataTypeStr=Inherit: Same as second input  aMode=0
  Sum : Sum  Inputs=|+-
  Uq_target : Outport
  wires:
  Fn_Target/1 -> Sum/1
  Sum/1 -> PID Controller/1
  PID Controller/1 -> Uq_target/1
  Fn_Actual/1 -> Sum/2

== system EMB_Lost_full/EMB_Ffl/Subsystem4 ==
  Speed_Actual : Inport
  S_Actual : Inport  Port=2
  PID Controller : slpidlib/PID Controller  Controller=PI  Form=Parallel  TimeDomain=Continuous-time  UseExternalTs=off  SampleTime=-1  IntegratorMethod=Forward Euler  FilterMethod=Forward Euler  ControllerParametersSource=internal  P=10000  I=0  UseKiTs=off  D=0  N=100  UseFilter=on  TunerSelectOption=Transfer Function Based (PID Tuner App)  InitialConditionSource=internal  InitialConditionForIntegrator=0  InitialConditionForFilter=0  DifferentiatorICPrevScaledInput=0  ExternalReset=none  TrackingMode=off  Kt=1  LimitOutput=on  SatLimitsSource=internal  UpperSaturationLimit=1000  LowerSaturationLimit=-1000  LinearizeAsGain=on  AntiWindupMode=none  Kb=1  POutMin=[]  POutMax=[]  IOutMin=[]  IOutMax=[]  DOutMin=[]  DOutMax=[]  NOutMin=[]  NOutMax=[]  SumOutMin=[]  SumOutMax=[]  SaturationOutMin=[]  SaturationOutMax=[]  PParamMin=[]  PParamMax=[]  IParamMin=[]  IParamMax=[]  DParamMin=[]  DParamMax=[]  NParamMin=[]  NParamMax=[]  KbParamMin=[]  KbParamMax=[]  KtParamMin=[]  KtParamMax=[]  KbOutMin=[]  KbOutMax=[]  KtOutMin=[]  KtOutMax=[]  IntegratorOutMin=[]  IntegratorOutMax=[]  FilterOutMin=[]  FilterOutMax=[]  SumI1OutMin=[]  SumI1OutMax=[]  SumI2OutMin=[]  SumI2OutMax=[]  SumI3OutMin=[]  SumI3OutMax=[]  SumI4OutMin=[]  SumI4OutMax=[]  SumDOutMin=[]  SumDOutMax=[]  DifferentiatorOutMin=[]  DifferentiatorOutMax=[]  FilterDiffOutCoefMin=[]  FilterDiffOutCoefMax=[]  ReciprocalOutMin=[]  ReciprocalOutMax=[]  SumDenOutMin=[]  SumDenOutMax=[]  SumNumOutMin=[]  SumNumOutMax=[]  DivideOutMin=[]  DivideOutMax=[]  UdiffTsProdOutMin=[]  UdiffTsProdOutMax=[]  NTsProdOutMin=[]  NTsProdOutMax=[]  UintegralTsProdOutMin=[]  UintegralTsProdOutMax=[]  UngainTsProdOutMin=[]  UngainTsProdOutMax=[]  IntegratorContinuousStateAttributes=''  IntegratorStateMustResolveToSignalObject=off  IntegratorRTWStateStorageClass=Auto  FilterContinuousStateAttributes=''  FilterStateMustResolveToSignalObject=off  FilterRTWStateStorageClass=Auto  ParallelPVariant=InternalParameters  IdealPVariant=Disabled  IVariant=InternalParameters  DVariant=Disabled  IntegratorVariant=Continuous  SatVariant=Enabled  AWVariant=Passthrough  PCopyVariant=Disabled  TRVariant=Disabled  FdbkBlocksVariant=Forward  IdealPFdbkVariant=Disabled  SatFdbkVariant=Disabled  DerivativeFilterVariant=Disabled  NVariant=Disabled  NCopyVariant=Disabled_SignalSpec  FilterICVariant=Disabled  IntegratorICVariant=InternalICs  ExternalResetVariant=Disabled  TRSumVariant=Passthrough  SumFdbkVariant=Disabled  SumVariant=Sum_PI  TsampFilterVariant=InternalTs  TsampNgainVariant=Passthrough  TsampIntegralVariant=Passthrough  ExternalSaturationOutDataTypeStr=Inherit: Same as second input  aMode=0
  PID Controller1 : slpidlib/PID Controller  Controller=PI  Form=Parallel  TimeDomain=Continuous-time  UseExternalTs=off  SampleTime=-1  IntegratorMethod=Forward Euler  FilterMethod=Forward Euler  ControllerParametersSource=internal  P=0.2  I=0  UseKiTs=off  D=0  N=100  UseFilter=on  TunerSelectOption=Transfer Function Based (PID Tuner App)  InitialConditionSource=internal  InitialConditionForIntegrator=0  InitialConditionForFilter=0  DifferentiatorICPrevScaledInput=0  ExternalReset=none  TrackingMode=off  Kt=1  LimitOutput=on  SatLimitsSource=internal  UpperSaturationLimit=24  LowerSaturationLimit=-24  LinearizeAsGain=on  AntiWindupMode=none  Kb=1  POutMin=[]  POutMax=[]  IOutMin=[]  IOutMax=[]  DOutMin=[]  DOutMax=[]  NOutMin=[]  NOutMax=[]  SumOutMin=[]  SumOutMax=[]  SaturationOutMin=[]  SaturationOutMax=[]  PParamMin=[]  PParamMax=[]  IParamMin=[]  IParamMax=[]  DParamMin=[]  DParamMax=[]  NParamMin=[]  NParamMax=[]  KbParamMin=[]  KbParamMax=[]  KtParamMin=[]  KtParamMax=[]  KbOutMin=[]  KbOutMax=[]  KtOutMin=[]  KtOutMax=[]  IntegratorOutMin=[]  IntegratorOutMax=[]  FilterOutMin=[]  FilterOutMax=[]  SumI1OutMin=[]  SumI1OutMax=[]  SumI2OutMin=[]  SumI2OutMax=[]  SumI3OutMin=[]  SumI3OutMax=[]  SumI4OutMin=[]  SumI4OutMax=[]  SumDOutMin=[]  SumDOutMax=[]  DifferentiatorOutMin=[]  DifferentiatorOutMax=[]  FilterDiffOutCoefMin=[]  FilterDiffOutCoefMax=[]  ReciprocalOutMin=[]  ReciprocalOutMax=[]  SumDenOutMin=[]  SumDenOutMax=[]  SumNumOutMin=[]  SumNumOutMax=[]  DivideOutMin=[]  DivideOutMax=[]  UdiffTsProdOutMin=[]  UdiffTsProdOutMax=[]  NTsProdOutMin=[]  NTsProdOutMax=[]  UintegralTsProdOutMin=[]  UintegralTsProdOutMax=[]  UngainTsProdOutMin=[]  UngainTsProdOutMax=[]  IntegratorContinuousStateAttributes=''  IntegratorStateMustResolveToSignalObject=off  IntegratorRTWStateStorageClass=Auto  FilterContinuousStateAttributes=''  FilterStateMustResolveToSignalObject=off  FilterRTWStateStorageClass=Auto  ParallelPVariant=InternalParameters  IdealPVariant=Disabled  IVariant=InternalParameters  DVariant=Disabled  IntegratorVariant=Continuous  SatVariant=Enabled  AWVariant=Passthrough  PCopyVariant=Disabled  TRVariant=Disabled  FdbkBlocksVariant=Forward  IdealPFdbkVariant=Disabled  SatFdbkVariant=Disabled  DerivativeFilterVariant=Disabled  NVariant=Disabled  NCopyVariant=Disabled_SignalSpec  FilterICVariant=Disabled  IntegratorICVariant=InternalICs  ExternalResetVariant=Disabled  TRSumVariant=Passthrough  SumFdbkVariant=Disabled  SumVariant=Sum_PI  TsampFilterVariant=InternalTs  TsampNgainVariant=Passthrough  TsampIntegralVariant=Passthrough  ExternalSaturationOutDataTypeStr=Inherit: Same as second input  aMode=0
  S_Target : Constant  Value=0
  Sum : Sum  Inputs=|+-
  Sum1 : Sum  Inputs=|+-
  Uq_target : Outport
  wires:
  S_Target/1 -> Sum/1
  Sum/1 -> PID Controller/1
  S_Actual/1 -> Sum/2
  PID Controller/1 -> Sum1/1
  Speed_Actual/1 -> Sum1/2
  PID Controller1/1 -> Uq_target/1
  Sum1/1 -> PID Controller1/1

== system EMB_Lost_full/EMB_Ffl/Ud_PI ==
  Ud_Target : Inport
  Ud_Actual : Inport  Port=2
  PID Controller : slpidlib/PID Controller  Controller=PI  Form=Parallel  TimeDomain=Continuous-time  UseExternalTs=off  SampleTime=-1  IntegratorMethod=Forward Euler  FilterMethod=Forward Euler  ControllerParametersSource=internal  P=0.12  I=0  UseKiTs=off  D=0.01  N=5  UseFilter=on  TunerSelectOption=Transfer Function Based (PID Tuner App)  InitialConditionSource=internal  InitialConditionForIntegrator=0  InitialConditionForFilter=0  DifferentiatorICPrevScaledInput=0  ExternalReset=none  TrackingMode=off  Kt=1  LimitOutput=on  SatLimitsSource=internal  UpperSaturationLimit=24  LowerSaturationLimit=-24  LinearizeAsGain=on  AntiWindupMode=none  Kb=1  POutMin=[]  POutMax=[]  IOutMin=[]  IOutMax=[]  DOutMin=[]  DOutMax=[]  NOutMin=[]  NOutMax=[]  SumOutMin=[]  SumOutMax=[]  SaturationOutMin=[]  SaturationOutMax=[]  PParamMin=[]  PParamMax=[]  IParamMin=[]  IParamMax=[]  DParamMin=[]  DParamMax=[]  NParamMin=[]  NParamMax=[]  KbParamMin=[]  KbParamMax=[]  KtParamMin=[]  KtParamMax=[]  KbOutMin=[]  KbOutMax=[]  KtOutMin=[]  KtOutMax=[]  IntegratorOutMin=[]  IntegratorOutMax=[]  FilterOutMin=[]  FilterOutMax=[]  SumI1OutMin=[]  SumI1OutMax=[]  SumI2OutMin=[]  SumI2OutMax=[]  SumI3OutMin=[]  SumI3OutMax=[]  SumI4OutMin=[]  SumI4OutMax=[]  SumDOutMin=[]  SumDOutMax=[]  DifferentiatorOutMin=[]  DifferentiatorOutMax=[]  FilterDiffOutCoefMin=[]  FilterDiffOutCoefMax=[]  ReciprocalOutMin=[]  ReciprocalOutMax=[]  SumDenOutMin=[]  SumDenOutMax=[]  SumNumOutMin=[]  SumNumOutMax=[]  DivideOutMin=[]  DivideOutMax=[]  UdiffTsProdOutMin=[]  UdiffTsProdOutMax=[]  NTsProdOutMin=[]  NTsProdOutMax=[]  UintegralTsProdOutMin=[]  UintegralTsProdOutMax=[]  UngainTsProdOutMin=[]  UngainTsProdOutMax=[]  IntegratorContinuousStateAttributes=''  IntegratorStateMustResolveToSignalObject=off  IntegratorRTWStateStorageClass=Auto  FilterContinuousStateAttributes=''  FilterStateMustResolveToSignalObject=off  FilterRTWStateStorageClass=Auto  ParallelPVariant=InternalParameters  IdealPVariant=Disabled  IVariant=InternalParameters  DVariant=Disabled  IntegratorVariant=Continuous  SatVariant=Enabled  AWVariant=Passthrough  PCopyVariant=Disabled  TRVariant=Disabled  FdbkBlocksVariant=Forward  IdealPFdbkVariant=Disabled  SatFdbkVariant=Disabled  DerivativeFilterVariant=Disabled  NVariant=Disabled  NCopyVariant=Disabled_SignalSpec  FilterICVariant=Disabled  IntegratorICVariant=InternalICs  ExternalResetVariant=Disabled  TRSumVariant=Passthrough  SumFdbkVariant=Disabled  SumVariant=Sum_PI  TsampFilterVariant=InternalTs  TsampNgainVariant=Passthrough  TsampIntegralVariant=Passthrough  ExternalSaturationOutDataTypeStr=Inherit: Same as second input  aMode=0
  Sum : Sum  Inputs=|+-
  Ud : Outport
  wires:
  Sum/1 -> PID Controller/1
  Ud_Actual/1 -> Sum/2
  Ud_Target/1 -> Sum/1
  PID Controller/1 -> Ud/1

== system EMB_Lost_full/EMB_Ffl/Uq_PI ==
  Uq_Target : Inport
  Uq_Actual : Inport  Port=2
  PID Controller : slpidlib/PID Controller  Controller=PI  Form=Parallel  TimeDomain=Continuous-time  UseExternalTs=off  SampleTime=-1  IntegratorMethod=Forward Euler  FilterMethod=Forward Euler  ControllerParametersSource=internal  P=0.12  I=0  UseKiTs=off  D=0.01  N=5  UseFilter=on  TunerSelectOption=Transfer Function Based (PID Tuner App)  InitialConditionSource=internal  InitialConditionForIntegrator=0  InitialConditionForFilter=0  DifferentiatorICPrevScaledInput=0  ExternalReset=none  TrackingMode=off  Kt=1  LimitOutput=on  SatLimitsSource=internal  UpperSaturationLimit=24  LowerSaturationLimit=-24  LinearizeAsGain=on  AntiWindupMode=none  Kb=1  POutMin=[]  POutMax=[]  IOutMin=[]  IOutMax=[]  DOutMin=[]  DOutMax=[]  NOutMin=[]  NOutMax=[]  SumOutMin=[]  SumOutMax=[]  SaturationOutMin=[]  SaturationOutMax=[]  PParamMin=[]  PParamMax=[]  IParamMin=[]  IParamMax=[]  DParamMin=[]  DParamMax=[]  NParamMin=[]  NParamMax=[]  KbParamMin=[]  KbParamMax=[]  KtParamMin=[]  KtParamMax=[]  KbOutMin=[]  KbOutMax=[]  KtOutMin=[]  KtOutMax=[]  IntegratorOutMin=[]  IntegratorOutMax=[]  FilterOutMin=[]  FilterOutMax=[]  SumI1OutMin=[]  SumI1OutMax=[]  SumI2OutMin=[]  SumI2OutMax=[]  SumI3OutMin=[]  SumI3OutMax=[]  SumI4OutMin=[]  SumI4OutMax=[]  SumDOutMin=[]  SumDOutMax=[]  DifferentiatorOutMin=[]  DifferentiatorOutMax=[]  FilterDiffOutCoefMin=[]  FilterDiffOutCoefMax=[]  ReciprocalOutMin=[]  ReciprocalOutMax=[]  SumDenOutMin=[]  SumDenOutMax=[]  SumNumOutMin=[]  SumNumOutMax=[]  DivideOutMin=[]  DivideOutMax=[]  UdiffTsProdOutMin=[]  UdiffTsProdOutMax=[]  NTsProdOutMin=[]  NTsProdOutMax=[]  UintegralTsProdOutMin=[]  UintegralTsProdOutMax=[]  UngainTsProdOutMin=[]  UngainTsProdOutMax=[]  IntegratorContinuousStateAttributes=''  IntegratorStateMustResolveToSignalObject=off  IntegratorRTWStateStorageClass=Auto  FilterContinuousStateAttributes=''  FilterStateMustResolveToSignalObject=off  FilterRTWStateStorageClass=Auto  ParallelPVariant=InternalParameters  IdealPVariant=Disabled  IVariant=InternalParameters  DVariant=Disabled  IntegratorVariant=Continuous  SatVariant=Enabled  AWVariant=Passthrough  PCopyVariant=Disabled  TRVariant=Disabled  FdbkBlocksVariant=Forward  IdealPFdbkVariant=Disabled  SatFdbkVariant=Disabled  DerivativeFilterVariant=Disabled  NVariant=Disabled  NCopyVariant=Disabled_SignalSpec  FilterICVariant=Disabled  IntegratorICVariant=InternalICs  ExternalResetVariant=Disabled  TRSumVariant=Passthrough  SumFdbkVariant=Disabled  SumVariant=Sum_PI  TsampFilterVariant=InternalTs  TsampNgainVariant=Passthrough  TsampIntegralVariant=Passthrough  ExternalSaturationOutDataTypeStr=Inherit: Same as second input  aMode=0
  Sum : Sum  Inputs=|+-
  Uq : Outport
  wires:
  Sum/1 -> PID Controller/1
  Uq_Actual/1 -> Sum/2
  PID Controller/1 -> Uq/1
  Uq_Target/1 -> Sum/1

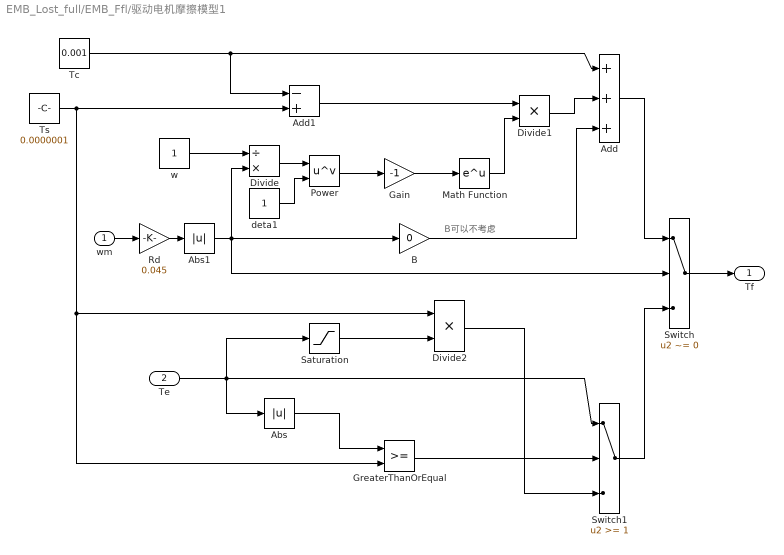
== system EMB_Lost_full/EMB_Ffl/驱动电机摩擦模型1 ==
  note: B可以不考虑
  wm : Inport
  Te : Inport  Port=2
  Abs : Abs  SaturateOnIntegerOverflow=off
  Abs1 : Abs  SaturateOnIntegerOverflow=off
  Add : Sum  Inputs=+++
  Add1 : Sum  Inputs=-+
  B : Gain  Gain=0
  Divide : Product  Inputs=/*
  Divide1 : Product  Inputs=**
  Divide2 : Product  Inputs=**
  Gain : Gain  Gain=-1
  GreaterThanOrEqual : RelationalOperator  OutDataTypeStr=boolean  RndMeth=Simplest  InputSameDT=off
  Math Function : Math
  Power : Math  Operator=pow
  Rd : Gain  Gain=0.045
  Saturation : Saturate  UpperLimit=1  LowerLimit=-1
  Switch : Switch  Criteria=u2 ~= 0  SaturateOnIntegerOverflow=off  InputSameDT=off
  Switch1 : Switch  Threshold=1  SaturateOnIntegerOverflow=off  InputSameDT=off
  Tc : Constant  Value=0.001
  Ts : Constant  Value=0.0000001
  deta1 : Constant
  w : Constant
  Tf : Outport
  wires:
  Tc/1 -> Add1/1, Add/1
  Ts/1 -> Add1/2, Divide2/1, GreaterThanOrEqual/2
  B/1 -> Add/3
  w/1 -> Divide/1
  Divide/1 -> Power/1
  deta1/1 -> Power/2
  Add1/1 -> Divide1/1
  Math Function/1 -> Divide1/2
  Divide1/1 -> Add/2
  Power/1 -> Gain/1
  Gain/1 -> Math Function/1
  Switch/1 -> Tf/1
  Add/1 -> Switch/1
  Switch1/1 -> Switch/3
  Te/1 -> Saturation/1, Switch1/1, Abs/1
  Abs/1 -> GreaterThanOrEqual/1
  GreaterThanOrEqual/1 -> Switch1/2
  Saturation/1 -> Divide2/2
  Divide2/1 -> Switch1/3
  wm/1 -> Rd/1
  Rd/1 -> Abs1/1
  Abs1/1 -> Switch/2, B/1, Divide/2

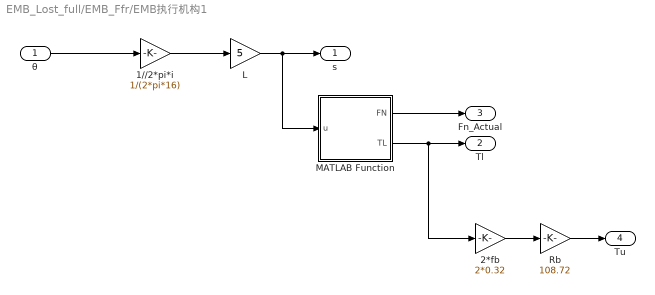
== system EMB_Lost_full/EMB_Ffr/EMB执行机构1 ==
  θ : Inport
  1//2*pi*i : Gain  Gain=1/(2*pi*16)
  2*fb : Gain  Gain=2*0.32
  L : Gain  Gain=5
  MATLAB Function : MATLAB Function  TreatAsAtomicUnit=on
  Rb : Gain  Gain=108.72
  s : Outport
  Tl : Outport  Port=2
  Fn_Actual : Outport  Port=3
  Tu : Outport  Port=4
  wires:
  θ/1 -> 1//2*pi*i/1
  1//2*pi*i/1 -> L/1
  L/1 -> MATLAB Function/1(u), s/1
  MATLAB Function/2(TL) -> 2*fb/1, Tl/1
  MATLAB Function/1(FN) -> Fn_Actual/1
  Rb/1 -> Tu/1
  2*fb/1 -> Rb/1

== system EMB_Lost_full/EMB_Ffr/EMB执行策略判断2 ==
  Fn_Target : Inport
  Fn_Actual : Inport  Port=2
  Fn_Threshold : Inport  Port=3
  MATLAB Function : MATLAB Function  TreatAsAtomicUnit=on
  sign : Outport
  wires:
  Fn_Target/1 -> MATLAB Function/1(Fn_Target)
  Fn_Actual/1 -> MATLAB Function/2(Fn_Actual)
  Fn_Threshold/1 -> MATLAB Function/3(Fn_Threshold)
  MATLAB Function/1(y) -> sign/1

== system EMB_Lost_full/EMB_Ffr/Subsystem2 ==
  Speed_Actual : Inport
  PID Controller : slpidlib/PID Controller  Controller=PI  Form=Parallel  TimeDomain=Continuous-time  UseExternalTs=off  SampleTime=-1  IntegratorMethod=Forward Euler  FilterMethod=Forward Euler  ControllerParametersSource=internal  P=1000  I=0  UseKiTs=off  D=0  N=100  UseFilter=on  TunerSelectOption=Transfer Function Based (PID Tuner App)  InitialConditionSource=internal  InitialConditionForIntegrator=0  InitialConditionForFilter=0  DifferentiatorICPrevScaledInput=0  ExternalReset=none  TrackingMode=off  Kt=1  LimitOutput=on  SatLimitsSource=internal  UpperSaturationLimit=24  LowerSaturationLimit=-24  LinearizeAsGain=on  AntiWindupMode=none  Kb=1  POutMin=[]  POutMax=[]  IOutMin=[]  IOutMax=[]  DOutMin=[]  DOutMax=[]  NOutMin=[]  NOutMax=[]  SumOutMin=[]  SumOutMax=[]  SaturationOutMin=[]  SaturationOutMax=[]  PParamMin=[]  PParamMax=[]  IParamMin=[]  IParamMax=[]  DParamMin=[]  DParamMax=[]  NParamMin=[]  NParamMax=[]  KbParamMin=[]  KbParamMax=[]  KtParamMin=[]  KtParamMax=[]  KbOutMin=[]  KbOutMax=[]  KtOutMin=[]  KtOutMax=[]  IntegratorOutMin=[]  IntegratorOutMax=[]  FilterOutMin=[]  FilterOutMax=[]  SumI1OutMin=[]  SumI1OutMax=[]  SumI2OutMin=[]  SumI2OutMax=[]  SumI3OutMin=[]  SumI3OutMax=[]  SumI4OutMin=[]  SumI4OutMax=[]  SumDOutMin=[]  SumDOutMax=[]  DifferentiatorOutMin=[]  DifferentiatorOutMax=[]  FilterDiffOutCoefMin=[]  FilterDiffOutCoefMax=[]  ReciprocalOutMin=[]  ReciprocalOutMax=[]  SumDenOutMin=[]  SumDenOutMax=[]  SumNumOutMin=[]  SumNumOutMax=[]  DivideOutMin=[]  DivideOutMax=[]  UdiffTsProdOutMin=[]  UdiffTsProdOutMax=[]  NTsProdOutMin=[]  NTsProdOutMax=[]  UintegralTsProdOutMin=[]  UintegralTsProdOutMax=[]  UngainTsProdOutMin=[]  UngainTsProdOutMax=[]  IntegratorContinuousStateAttributes=''  IntegratorStateMustResolveToSignalObject=off  IntegratorRTWStateStorageClass=Auto  FilterContinuousStateAttributes=''  FilterStateMustResolveToSignalObject=off  FilterRTWStateStorageClass=Auto  ParallelPVariant=InternalParameters  IdealPVariant=Disabled  IVariant=InternalParameters  DVariant=Disabled  IntegratorVariant=Continuous  SatVariant=Enabled  AWVariant=Passthrough  PCopyVariant=Disabled  TRVariant=Disabled  FdbkBlocksVariant=Forward  IdealPFdbkVariant=Disabled  SatFdbkVariant=Disabled  DerivativeFilterVariant=Disabled  NVariant=Disabled  NCopyVariant=Disabled_SignalSpec  FilterICVariant=Disabled  IntegratorICVariant=InternalICs  ExternalResetVariant=Disabled  TRSumVariant=Passthrough  SumFdbkVariant=Disabled  SumVariant=Sum_PI  TsampFilterVariant=InternalTs  TsampNgainVariant=Passthrough  TsampIntegralVariant=Passthrough  ExternalSaturationOutDataTypeStr=Inherit: Same as second input  aMode=0
  Speed_Target : Constant  Value=1000
  Sum : Sum  Inputs=|+-
  Uq_target : Outport
  wires:
  Speed_Target/1 -> Sum/1
  Sum/1 -> PID Controller/1
  PID Controller/1 -> Uq_target/1
  Speed_Actual/1 -> Sum/2
